simulink model "Laba_1Timchenko"  (Simulink 6.6)
settings: Solver=ode45  StartTime=0.0  StopTime=0.4  RelTol=1e-3
settings Model: Creator=student  LastModifiedBy=student
settings DataIOCC: SignalLoggingName=sigsOut
settings DebuggingCC: SignalResolutionControl=TryResolveAllWithWarning  SolverPrmCheckMsg=none  MultiTaskDSMMsg=warning  MultiTaskCondExecSysMsg=none  StrictBusMsg=None
settings HardwareCC: TargetUnknown=on
settings RTWCC: IncludeERTFirstTime=on

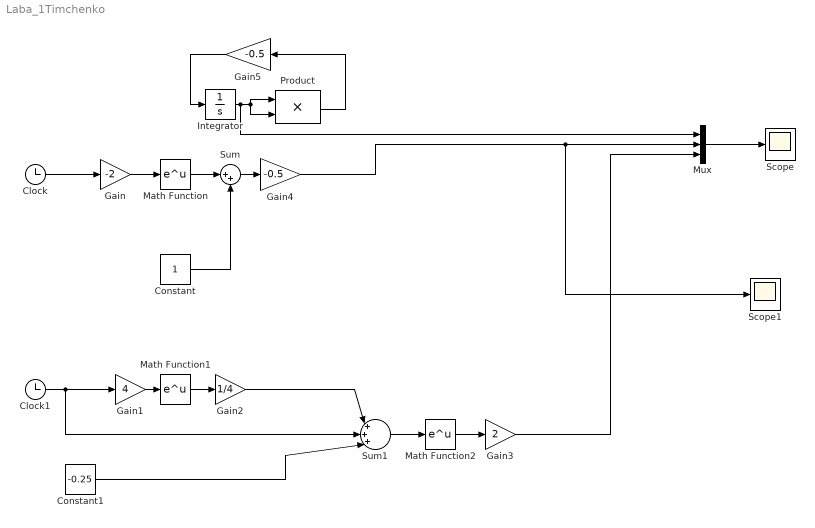
== system Laba_1Timchenko ==
  Clock : Clock
      settings: Decimation=10
  Clock1 : Clock
      settings: Decimation=4
  Constant : Constant
  Constant1 : Constant  Value=-0.25
  Gain : Gain  Gain=-2  SaturateOnIntegerOverflow=on
  Gain1 : Gain  Gain=4  SaturateOnIntegerOverflow=on
  Gain2 : Gain  Gain=1/4  SaturateOnIntegerOverflow=on
  Gain3 : Gain  Gain=2  SaturateOnIntegerOverflow=on
  Gain4 : Gain  Gain=-0.5
  Gain5 : Gain  Orientation=left  Gain=-0.5  SaturateOnIntegerOverflow=on
  Integrator : Integrator  InitialCondition=2
  Math Function : Math  SaturateOnIntegerOverflow=on
  Math Function1 : Math  SaturateOnIntegerOverflow=on
  Math Function2 : Math  SaturateOnIntegerOverflow=on
  Mux : Mux  Inputs=3
  Product : Product  SaturateOnIntegerOverflow=on
  Scope : Scope
  Scope1 : Scope
  Sum : Sum  Inputs=|++  SaturateOnIntegerOverflow=on
  Sum1 : Sum  Inputs=|+++|  SaturateOnIntegerOverflow=on
  wires:
  Integrator/1 -> Product/1, Product/2, Mux/1
  Product/1 -> Gain5/1
  Clock/1 -> Gain/1
  Gain/1 -> Math Function/1
  Math Function/1 -> Sum/1
  Constant/1 -> Sum/2
  Sum/1 -> Gain4/1
  Mux/1 -> Scope/1
  Gain1/1 -> Math Function1/1
  Math Function1/1 -> Gain2/1
  Gain2/1 -> Sum1/1
  Clock1/1 -> Gain1/1, Sum1/2
  Constant1/1 -> Sum1/3
  Sum1/1 -> Math Function2/1
  Math Function2/1 -> Gain3/1
  Gain3/1 -> Mux/3
  Gain4/1 -> Mux/2, Scope1/1
  Gain5/1 -> Integrator/1
